simulink model "threeBodyProblem"  (R2025b)
settings: Solver=ode45  StartTime=0.0  StopTime=20  MaxStep=0.01  RelTol=1e-3
settings Model: Creator=mizula  LastModifiedBy=mizula

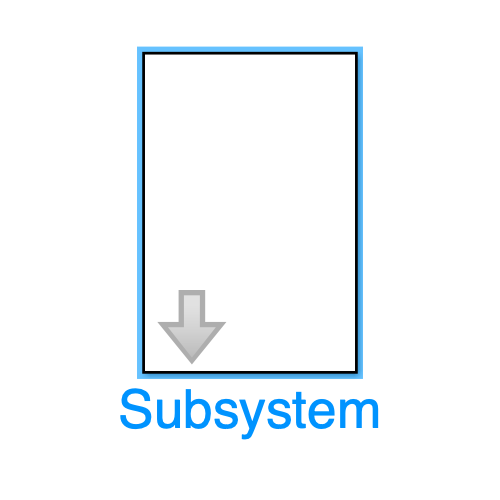
[thumbnail: Simulink's stored preview of the top-level diagram]
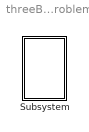
== system threeBodyProblem ==
  Subsystem : Subsystem  mask{G=1, m1=3, m2=1, m3=1, x10=0.97000436, y10=-0.24308753, vx10=0.466203685, vy10=0.43236573, x20=0, y20=0, vx20=-0.93240737, vy20=-0.86473146, x30=-0.97000436, y30=0.24308753, vx30=0.466203685, vy30=0.43236573}

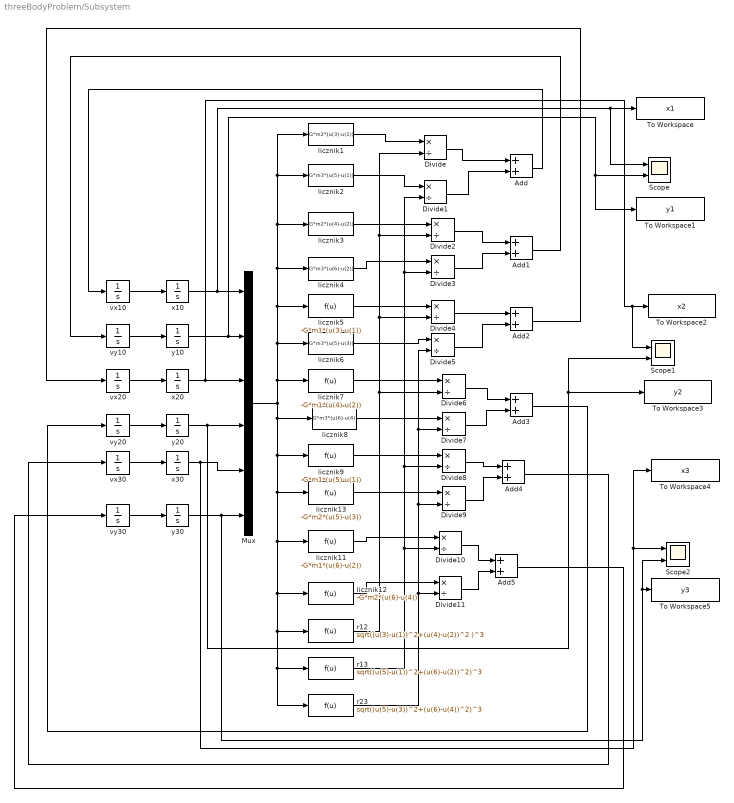
== system threeBodyProblem/Subsystem ==
  Add{,1..5} (6 alike) : Sum
  Divide{,1..11} (12 alike) : Product  Inputs=*/
  Mux : Mux  Inputs=6
  Scope : Scope  NumInputPorts=2
      settings: ActiveDisplayYMinimum=-1  ActiveDisplayYMaximum=1
  Scope1 : Scope  NumInputPorts=2
      settings: ActiveDisplayYMinimum=-1  ActiveDisplayYMaximum=1
  Scope2 : Scope  NumInputPorts=2
      settings: ActiveDisplayYMinimum=-1.4838811315334593E+10  ActiveDisplayYMaximum=8.6390749466036549E+9  DataLoggingVariableName=ScopeData2
  To Workspace : ToWorkspace  VariableName=x1  SaveFormat=Timeseries  SampleTime=-1
  To Workspace1 : ToWorkspace  VariableName=y1  SaveFormat=Timeseries  SampleTime=-1
  To Workspace2 : ToWorkspace  VariableName=x2  SaveFormat=Timeseries  SampleTime=-1
  To Workspace3 : ToWorkspace  VariableName=y2  SaveFormat=Timeseries  SampleTime=-1
  To Workspace4 : ToWorkspace  VariableName=x3  SaveFormat=Timeseries  SampleTime=-1
  To Workspace5 : ToWorkspace  VariableName=y3  SaveFormat=Timeseries  SampleTime=-1
  licznik1 : Fcn  Expr=G*m2*(u(3)-u(1))
  licznik11 : Fcn  Expr=-G*m1*(u(6)-u(2))
  licznik12 : Fcn  Expr=-G*m2*(u(6)-u(4))
  licznik13 : Fcn  Expr=-G*m2*(u(5)-u(3))
  licznik2 : Fcn  Expr=G*m3*(u(5)-u(1))
  licznik3 : Fcn  Expr=G*m2*(u(4)-u(2))
  licznik4 : Fcn  Expr=G*m3*(u(6)-u(2))
  licznik5 : Fcn  Expr=-G*m1*(u(3)-u(1))
  licznik6 : Fcn  Expr=G*m3*(u(5)-u(3))
  licznik7 : Fcn  Expr=-G*m1*(u(4)-u(2))
  licznik8 : Fcn  Expr=G*m3*(u(6)-u(4))
  licznik9 : Fcn  Expr=-G*m1*(u(5)-u(1))
  r12 : Fcn  Expr=sqrt((u(3)-u(1))^2+(u(4)-u(2))^2 )^3
  r13 : Fcn  Expr=sqrt((u(5)-u(1))^2+(u(6)-u(2))^2)^3
  r23 : Fcn  Expr=sqrt((u(5)-u(3))^2+(u(6)-u(4))^2)^3
  vx10 : Integrator  InitialCondition=vx10
  vx20 : Integrator  InitialCondition=vx20
  vx30 : Integrator  InitialCondition=vx30
  vy10 : Integrator  InitialCondition=vy10
  vy20 : Integrator  InitialCondition=vy20
  vy30 : Integrator  InitialCondition=vy30
  x10 : Integrator  InitialCondition=x10
  x20 : Integrator  InitialCondition=x20
  x30 : Integrator  InitialCondition=x30
  y10 : Integrator  InitialCondition=y10
  y20 : Integrator  InitialCondition=y20
  y30 : Integrator  InitialCondition=y30
  wires:
  vx10/1 -> x10/1
  vy10/1 -> y10/1
  vx20/1 -> x20/1
  vy20/1 -> y20/1
  vx30/1 -> x30/1
  vy30/1 -> y30/1
  x10/1 -> Scope/1, To Workspace/1, Mux/1
  y10/1 -> To Workspace1/1, Scope/2, Mux/2
  x20/1 -> Scope1/1, To Workspace2/1, Mux/3
  y20/1 -> Mux/4, Scope1/2, To Workspace3/1
  x30/1 -> To Workspace4/1, Scope2/1, Mux/5
  y30/1 -> To Workspace5/1, Scope2/2, Mux/6
  Mux/1 -> licznik9/1, licznik13/1, licznik11/1, licznik12/1, r12/1, r13/1, r23/1, licznik8/1, licznik7/1, licznik6/1, licznik5/1, licznik4/1, licznik3/1, licznik2/1, licznik1/1
  licznik1/1 -> Divide/1
  r12/1 -> Divide6/2, Divide/2, Divide2/2, Divide4/2
  licznik2/1 -> Divide1/1
  r13/1 -> Divide10/2, Divide3/2, Divide1/2, Divide8/2
  Divide/1 -> Add/1
  Divide1/1 -> Add/2
  licznik3/1 -> Divide2/1
  licznik4/1 -> Divide3/1
  Divide2/1 -> Add1/1
  Divide3/1 -> Add1/2
  licznik5/1 -> Divide4/1
  licznik6/1 -> Divide5/1
  r23/1 -> Divide7/2, Divide5/2, Divide9/2, Divide11/2
  Divide4/1 -> Add2/1
  Divide5/1 -> Add2/2
  licznik7/1 -> Divide6/1
  licznik8/1 -> Divide7/1
  Divide6/1 -> Add3/1
  Divide7/1 -> Add3/2
  licznik9/1 -> Divide8/1
  licznik13/1 -> Divide9/1
  Divide8/1 -> Add4/1
  Divide9/1 -> Add4/2
  licznik11/1 -> Divide10/1
  licznik12/1 -> Divide11/1
  Divide10/1 -> Add5/1
  Divide11/1 -> Add5/2
  Add/1 -> vx10/1
  Add1/1 -> vy10/1
  Add2/1 -> vx20/1
  Add3/1 -> vy20/1
  Add4/1 -> vx30/1
  Add5/1 -> vy30/1
